simulink model "ElectromechanicalProblem_Sim_interpolation"  (R2020b)
settings: Solver=VariableStepAuto  StartTime=0.0  StopTime=1  MaxStep=10^-3  RelTol=1e-3
values from neighbouring files (symbols this model uses):
  c = 0.5    [ElectromechanicalProblem.m]    (also in ElectromechanicalProblem_interpolation.m)
  i = linspace(0.001,6,np).'    [ElectromechanicalProblem_interpolation.m]
  k = 10000    [ElectromechanicalProblem.m]    (also in ElectromechanicalProblem_interpolation.m)
  L_s = 0    [ElectromechanicalProblem.m]    (also in ElectromechanicalProblem_interpolation.m)
  m = 2    [ElectromechanicalProblem.m]    (also in ElectromechanicalProblem_interpolation.m)
  R_m = 1.8833    [ElectromechanicalProblem.m]    (also in ElectromechanicalProblem_interpolation.m)
  R_s = 0    [ElectromechanicalProblem.m]    (also in ElectromechanicalProblem_interpolation.m)
  V_s = 10    [ElectromechanicalProblem.m]    (also in ElectromechanicalProblem_interpolation.m)
  x = linspace(0.005,0.03,np).'    [ElectromechanicalProblem_interpolation.m]
  x0 = 0.02    [ElectromechanicalProblem.m]    (also in ElectromechanicalProblem_interpolation.m)
undefined symbols (not defined in the file or in its folder): F_input, lamda_di, lamda_dx, lamda_input
settings Model: Creator=claud  LastModifiedBy=claud

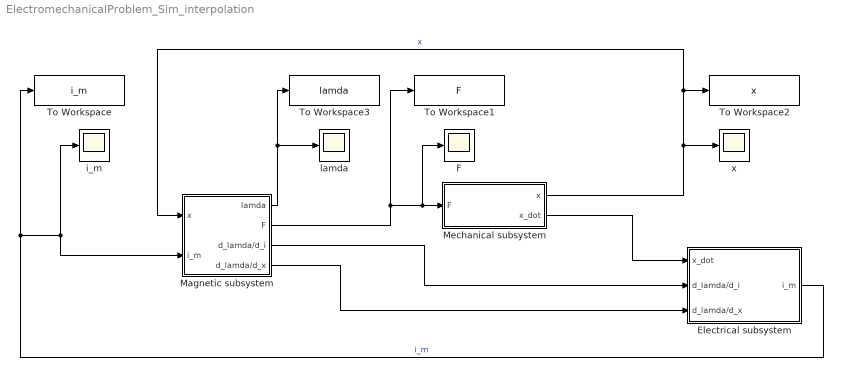
== system ElectromechanicalProblem_Sim_interpolation ==
  Electrical subsystem : Subsystem
  F : Scope
  Magnetic subsystem : Subsystem
  Mechanical subsystem : Subsystem
  To Workspace : ToWorkspace  VariableName=i_m  SaveFormat=Timeseries  SampleTime=-1
  To Workspace1 : ToWorkspace  VariableName=F  SaveFormat=Timeseries  SampleTime=-1
  To Workspace2 : ToWorkspace  VariableName=x  SaveFormat=Timeseries  SampleTime=-1
  To Workspace3 : ToWorkspace  VariableName=lamda  SaveFormat=Timeseries  SampleTime=-1
  i_m : Scope
  lamda : Scope
  x : Scope
  wires:
  Mechanical subsystem/1(x) -> To Workspace2/1, Magnetic subsystem/1(x), x/1  "x"
  Electrical subsystem/1(i_m) -> To Workspace/1, i_m/1, Magnetic subsystem/2(i_m)  "i_m"
  Magnetic subsystem/2(F) -> To Workspace1/1, F/1, Mechanical subsystem/1(F)
  Mechanical subsystem/2(x_dot) -> Electrical subsystem/1(x_dot)
  Magnetic subsystem/3(d_lamda/d_i) -> Electrical subsystem/2(d_lamda/d_i)
  Magnetic subsystem/4(d_lamda/d_x) -> Electrical subsystem/3(d_lamda/d_x)
  Magnetic subsystem/1(lamda) -> To Workspace3/1, lamda/1

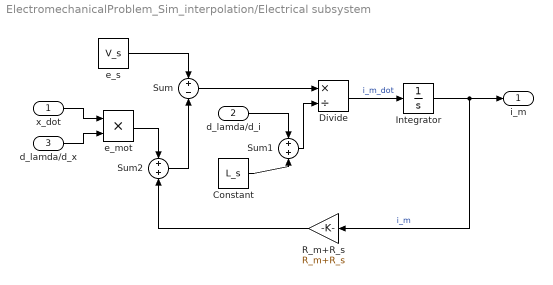
== system ElectromechanicalProblem_Sim_interpolation/Electrical subsystem ==
  x_dot : Inport
  d_lamda/d_i : Inport  Port=2
  d_lamda/d_x : Inport  Port=3
  Constant : Constant  Value=L_s
  Divide : Product  Inputs=*/
  Integrator : Integrator
  R_m+R_s : Gain  Gain=R_m+R_s
  Sum : Sum  Inputs=+-
  Sum1 : Sum
  Sum2 : Sum
  e_mot : Product
  e_s : Constant  Value=V_s
  i_m : Outport
  wires:
  e_s/1 -> Sum/1
  Constant/1 -> Sum1/2
  Sum1/1 -> Divide/2
  Sum/1 -> Divide/1
  Divide/1 -> Integrator/1  "i_m_dot"
  Integrator/1 -> R_m+R_s/1, i_m/1  "i_m"
  d_lamda/d_i/1 -> Sum1/1
  R_m+R_s/1 -> Sum2/2
  Sum2/1 -> Sum/2
  e_mot/1 -> Sum2/1
  x_dot/1 -> e_mot/1
  d_lamda/d_x/1 -> e_mot/2

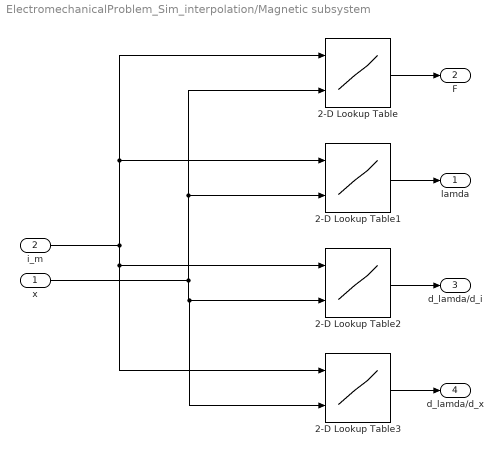
== system ElectromechanicalProblem_Sim_interpolation/Magnetic subsystem ==
  x : Inport
  i_m : Inport  Port=2
  2-D Lookup Table : Lookup_n-D  BreakpointsForDimension1=i  BreakpointsForDimension2=x  BreakpointsForDimension3Source=Input port  Table=F_input  InternalRulePriority=Speed  RndMeth=Simplest  InputSameDT=on
      settings: InputPortMap=u0,u1
  2-D Lookup Table1 : Lookup_n-D  BreakpointsForDimension1=i  BreakpointsForDimension2=x  BreakpointsForDimension3Source=Input port  Table=lamda_input  InternalRulePriority=Speed  RndMeth=Simplest  InputSameDT=on
      settings: InputPortMap=u0,u1
  2-D Lookup Table2 : Lookup_n-D  BreakpointsForDimension1=i  BreakpointsForDimension2=x  BreakpointsForDimension3Source=Input port  Table=lamda_di  InternalRulePriority=Speed  RndMeth=Simplest  InputSameDT=on
      settings: InputPortMap=u0,u1
  2-D Lookup Table3 : Lookup_n-D  BreakpointsForDimension1=i  BreakpointsForDimension2=x  BreakpointsForDimension3Source=Input port  Table=lamda_dx  InternalRulePriority=Speed  RndMeth=Simplest  InputSameDT=on
      settings: InputPortMap=u0,u1
  lamda : Outport
  F : Outport  Port=2
  d_lamda/d_i : Outport  Port=3
  d_lamda/d_x : Outport  Port=4
  wires:
  2-D Lookup Table/1 -> F/1
  2-D Lookup Table1/1 -> lamda/1
  2-D Lookup Table2/1 -> d_lamda/d_i/1
  i_m/1 -> 2-D Lookup Table1/1, 2-D Lookup Table/1, 2-D Lookup Table3/1, 2-D Lookup Table2/1
  x/1 -> 2-D Lookup Table1/2, 2-D Lookup Table/2, 2-D Lookup Table3/2, 2-D Lookup Table2/2
  2-D Lookup Table3/1 -> d_lamda/d_x/1

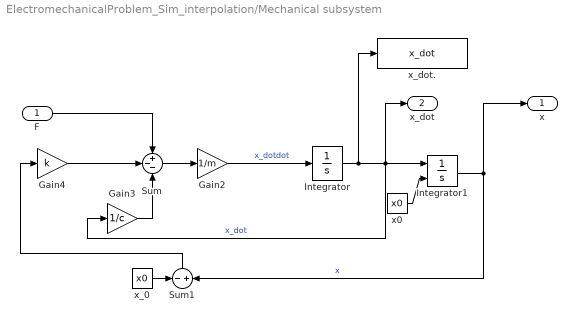
== system ElectromechanicalProblem_Sim_interpolation/Mechanical subsystem ==
  F : Inport
  Gain2 : Gain  Gain=1/m
  Gain3 : Gain  Gain=1/c
  Gain4 : Gain  Gain=k
  Integrator : Integrator
  Integrator1 : Integrator  InitialConditionSource=external  InitialCondition=0.02
  Sum : Sum  Inputs=+--
  Sum1 : Sum  Inputs=-+
  x0 : Constant  Value=x0
  x_0 : Constant  Value=x0
  x_dot. : ToWorkspace  VariableName=x_dot  SaveFormat=Timeseries  SampleTime=-1
  x : Outport
  x_dot : Outport  Port=2
  wires:
  Sum/1 -> Gain2/1
  Gain3/1 -> Sum/3
  Gain2/1 -> Integrator/1  "x_dotdot"
  F/1 -> Sum/1
  Gain4/1 -> Sum/2
  Integrator/1 -> Gain3/1, x_dot/1, Integrator1/1, x_dot./1  "x_dot"
  Integrator1/1 -> x/1, Sum1/2  "x"
  x0/1 -> Integrator1/2
  Sum1/1 -> Gain4/1
  x_0/1 -> Sum1/1
